simulink model "dng_bounce_subsys"  (Simulink 5.0)
settings: Solver=ode23  SolverMode=SingleTasking  StartTime=0.0  StopTime=20  MaxStep=.01  RelTol=1e-3  AbsTol=1e-6
libraries: dnglibv1 x4
settings Model: CovMetricSettings=d  Creator=monteiro  LastModifiedBy=howie  ExtModeTrigMode=oneshot  ExtModeArmWhenConnect=off  ExternalInput=[]  InitialState=[]  SaveTime=off  SaveOutput=off  LimitDataPoints=off  BlockReductionOpt=off  BooleanDataType=off

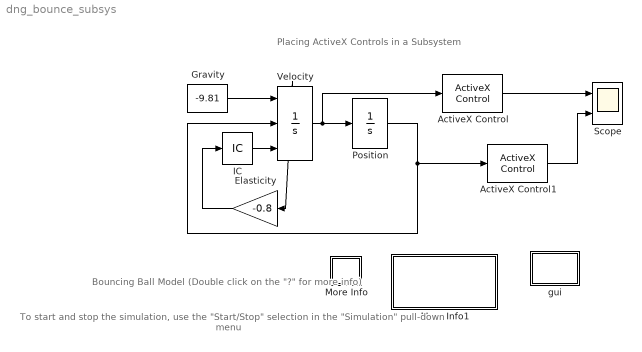
== system dng_bounce_subsys ==
  note: To start and stop the simulation, use the "Start/Stop"
      | selection in the "Simulation" pull-down menu
  note: Bouncing Ball Model
      | (Double click on the "?" for more info)
  note: Placing ActiveX Controls in a Subsystem
  ActiveX Control : dnglibv1/ActiveX Control  Tag=010  connect=both  input=NeedleValue  output=NeedleValue  init_fcn=dng_bounce_subsys/gui/Velocity  inblock=off  border=on  dialOut=0  updateParam=0
  ActiveX Control1 : dnglibv1/ActiveX Control  Tag=000  connect=both  input=PointerValue  output=PointerValue  init_fcn=dng_bounce_subsys/gui/Position  inblock=off  border=on  dialOut=0  updateParam=0
  Elasticity : Gain  Orientation=left  Gain=-0.8  SaturateOnIntegerOverflow=on
  Gravity : Constant  Value=-9.81
  IC : InitialCondition  Value=15
  More Info : Subsystem
      mask Display: disp('?')
  More Info1 : Subsystem
      settings: OpenFcn=simcad(bdroot);
      mask Display: disp('Double click\nhere for\nSimulink Help')
  Position : Integrator  InitialCondition=10  LimitOutput=on  LowerSaturationLimit=0
  Scope : Scope  NumInputPorts=2
      settings: TickLabels=on  TimeRange=20  YMin=-30~0  YMax=20~22.9822  DataFormat=Array
  Velocity : Integrator  ExternalReset=falling  InitialConditionSource=external  ShowStatePort=on
  gui : Subsystem
  wires:
  Velocity/State -> Elasticity/1
  IC/1 -> Velocity/3
  Elasticity/1 -> IC/1
  Velocity/1 -> Position/1, ActiveX Control/1
  Position/1 -> Velocity/2, ActiveX Control1/1
  Gravity/1 -> Velocity/1
  ActiveX Control/1 -> Scope/1
  ActiveX Control1/1 -> Scope/2

== system dng_bounce_subsys/More Info ==
  note: A rubber ball is thrown into the air with the velocity 15
      | meters per second from a height of 10 m.  The position
      |  of the ball is shown in the Bouncing Ball Display.
      | To view the velocity, double click on the Velocity Scope.
  note: This system uses a reset-integrator to change the
      | direction of the ball as it comes into contact with
      | the ground

== system dng_bounce_subsys/More Info1 ==

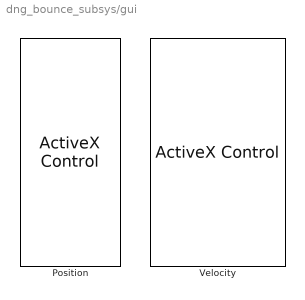
== system dng_bounce_subsys/gui ==
  Position : dnglibv1/ActiveX Control  progid=mwlgauge.lgaugectrl.1  connect=neither  inblock=on  border=on  dialOut=0  updateParam=0
  Velocity : dnglibv1/ActiveX Control  progid=mwagauge.agaugectrl.1  connect=neither  init=hActx.configuration='Angular Gauge\General Meters\Amp Meter';  inblock=on  border=on  dialOut=0  updateParam=0
